simulink library "buildingEnergyComposite"  (R2025b)
settings: Solver=VariableStepAuto  StartTime=0.0  StopTime=10.0  RelTol=1e-3
libraries: fl_lib x59, buildingEnergy_lib x9, SimscapeFluids_lib x1
settings Model: Creator=vikrants  LastModifiedBy=skota

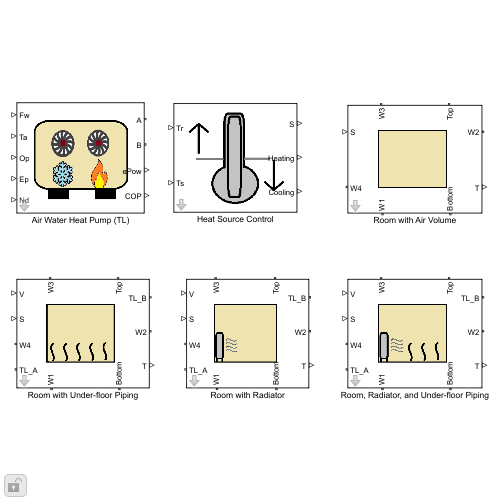
[thumbnail: Simulink's stored preview of the top-level diagram]
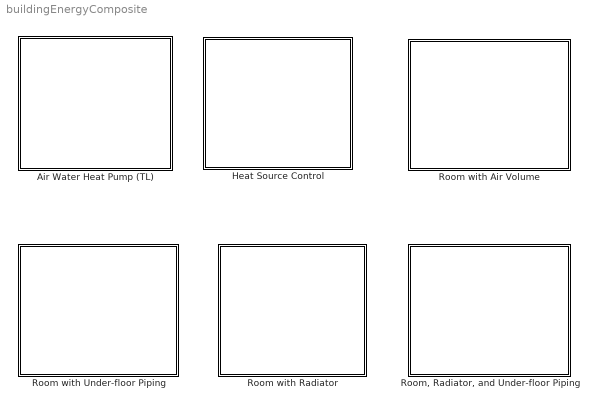
== system buildingEnergyComposite ==
  Air Water Heat Pump (TL) : Subsystem  mask{heatingCapacityA=10.17, heatingCoPA=4.86, heatingCapacityB=10.12, heatingCoPB=3.7, heatingCapacityC=10.17, heatingCoPC=4.86, heatingCapacityD=10.12, heatingCoPD=3.7, coolingCapacityE=10.55, coolingCoPE=4.13, coolingCapacityF=6.9, coolingCoPF=2.7, elecHeaterPower=0, coilLen=2, coilArea=pi*(5e-2^2)/4, coilDia=5e-2, tankVolume=5, initialT=299.8, waterOpTempMax=330, waterOpTempMin=278, initialP=0.101325, measTimelagWater=60, minWaterFlowRate=1e-3, nomFlowDuringTest=0.5}
      mask prompts: heatingCapacityA "A-2W55, estimated heating capacity (kW)"; heatingCoPA "A-2W55, estimated COP (or SCOP)"; heatingCapacityB "A-2W65, estimated heating capacity (kW)"; heatingCoPB "A-2W65, estimated COP (or SCOP)"; heatingCapacityC "A7W35, estimated heating capacity (kW)"; heatingCoPC "A7W35, estimated COP (or SCOP)"; heatingCapacityD "A7W45, estimated heating capacity (kW)"; heatingCoPD "A7W45, estimated COP (or SCOP)"; coolingCapacityE "A35W18, estimated cooling capacity (kW)"; coolingCoPE "A35W18, estimated COP (or SCOP)"; coolingCapacityF "A35W7, estimated cooling capacity (kW)"; coolingCoPF "A35W7, estimated COP (or SCOP)"; elecHeaterPower "Additional electric heater rating (kW)"; coilLen "Length of coil pipe (m)"; coilArea "Area of coil pipe (m^2)"; coilDia "Diameter of coil pipe (m)"; tankVolume "Heat exchanger internal volume (m^3)"; initialT "Initial Temperature (K)"; waterOpTempMax "Maximum operational water temperature"; waterOpTempMin "Minimum operation water temperature"; initialP "Initial pressure of coil pipe water (MPa)"; measTimelagWater "Temperature sensor delay for water flow (s)"; minWaterFlowRate "Minimum water flowrate (kg/s)"; nomFlowDuringTest "Nominal water flowrate during test (kg/s)"
      mask Help: web("DocumentationAirWaterHeatPumpTL.html")
      mask DialogControl DescGroupVar Prompt: Description
      mask DialogControl DescTextVar Prompt: Heat pump model based on EN14511 test data.
      mask DialogControl Container3 Prompt: EN14511 (Heating) Data
      mask DialogControl Container4 Prompt: EN14511 (Cooling) Data
      mask DialogControl ParameterGroupVar Prompt: Heat Pump Construction
      mask DialogControl Container5 Prompt: Flow and Thermal Specifications
      mask Display: image('AirWaterHeatPumpTL.png');
  Heat Source Control : Subsystem  mask{capacity=12000, num=1, delT=10, tau=1, iniT=280}
      mask prompts: capacity "Heat pump capacity (W)"; num "Number of sources (-)"; delT "Change in water temperature (deg C)"; tau "Measurement time constant (s)"; iniT "Initial water temperature (K)"
      mask Help: web("DocumentationCompositeHeatSourceControl.html")
      mask DialogControl DescGroupVar Prompt: Description
      mask DialogControl DescTextVar Prompt: The block evaluates heating or cooling requirements for a building  based on the measured room temperatures and the specified set point temperature.
      mask DialogControl HeatPump Prompt: Heat Pump
      mask Display: image('HeatSourceControlIcon.png');
  Room with Air Volume : Subsystem  mask{roomWid=3, roomHgt=2.5, roomLen=5, htc=10, iniT=300, indxS=1}
      mask prompts: roomWid "Room Width (m)"; roomHgt "Room Height (m)"; roomLen "Room Length (m)"; htc "Heat Transfer Coefficient (W/K*m^2)"; iniT "Initial Temperature (K)"; indxS "Heat source vector index"
      settings: PortSchema="{\"entries\":[{\"content\":{\"sides\":[{\"content\":{\"connectorIds\":[\"LConn1\",\"LConn2\"]},\"type\":\"ConnectorPlacement.EquallySpacedRectSide\",\"uuid\":\"8440f6ae-3089-4f14-af97-f7a7d9c670fb\"},{\"content\":{\"connectorIds\":[\"RConn1\",\"RConn2\"],\"side\":\"RIGHT\"},\"type\":\"ConnectorPlacement.EquallySpacedRectSide\",\"uuid\":\"df84a625-bd6d-46a4-b71c-d411d28f8df6\"},{\"content\":{\"connectorIds\":[\"LConn3\",\"LConn4\"],\"side\":\"TOP\"},\"type\":\"ConnectorPlacement.EquallySpacedRectSide\",\"uuid\":\"90f16a0a-d00c-4f13-8e79-f2f23ea8b565\"},{\"content\":{\"connectorIds\":[\"RConn3\",\"RConn4\"],\"side\":\"BOTTOM\"},\"type\":\"ConnectorPlacement.EquallySpacedRectSide\",\"uuid\":\"4eb9d9d9-e9b4-43a3-a1e1-726815f3b9ff\"}]},\"type\":\"ConnectorPlacement.EquallySpacedConnector\",\"uuid\":\"51dc529f-94b8-407e-b287-301b2c0c8383\"}],\"packageUris\":[\"http://schema.mathworks.com/mf0/Connector/R2020b\"],\"version\":\"1.0\"}"
      mask Help: web("DocumentationCompositeRoom.html")
      mask DialogControl DescGroupVar Prompt: Description
      mask DialogControl DescTextVar Prompt: Room model with air volume.
      mask DialogControl ParameterGroupRoom Prompt: Room Dimensions
      mask DialogControl ParameterGroupHT Prompt: Heat Transfer
      mask Display: image("roomWithAirVolume.png");
  Room with Radiator : Subsystem  mask{pipeRoughnessR=1e-6, pipeLenR=10, pipeCrossSectionalAreaR=1.75e-4, pipeHydrDiaR=1.5e-2, roomWid=3, roomHgt=2.5, roomLen=5, htc=10, iniT=300, indxS=1, indxV=1}
      mask prompts: pipeRoughnessR "Pipe roughness (m)"; pipeLenR "Pipe length (m)"; pipeCrossSectionalAreaR "Pipe cross-sectional area (m^2)"; pipeHydrDiaR "Pipe hydraulic diameter (m)"; roomWid "Room Width (m)"; roomHgt "Room Height (m)"; roomLen "Room Length (m)"; htc "Heat Transfer Coefficient (W/K*m^2)"; iniT "Initial Temperature (K)"; indxS "Heat source vector index"; indxV "Valve operation vector index"
      settings: PortSchema="{\"entries\":[{\"content\":{\"sides\":[{\"content\":{\"connectorIds\":[\"LConn1\",\"LConn2\",\"LConn3\",\"LConn4\"]},\"type\":\"ConnectorPlacement.EquallySpacedRectSide\",\"uuid\":\"8440f6ae-3089-4f14-af97-f7a7d9c670fb\"},{\"content\":{\"connectorIds\":[\"RConn1\",\"RConn2\",\"RConn3\"],\"side\":\"RIGHT\"},\"type\":\"ConnectorPlacement.EquallySpacedRectSide\",\"uuid\":\"df84a625-bd6d-46a4-b71c-d411d28f8df6\"},{\"content\":{\"connectorIds\":[\"LConn5\",\"LConn6\"],\"side\":\"TOP\"},\"type\":\"ConnectorPlacement.EquallySpacedRectSide\",\"uuid\":\"90f16a0a-d00c-4f13-8e79-f2f23ea8b565\"},{\"content\":{\"connectorIds\":[\"RConn4\",\"RConn5\"],\"side\":\"BOTTOM\"},\"type\":\"ConnectorPlacement.EquallySpacedRectSide\",\"uuid\":\"4eb9d9d9-e9b4-43a3-a1e1-726815f3b9ff\"}]},\"type\":\"ConnectorPlacement.EquallySpacedConnector\",\"uuid\":\"51dc529f-94b8-407e-b287-301b2c0c8383\"}],\"packageUris\":[\"http://schema.mathworks.com/mf0/Connector/R2020b\"],\"version\":\"1.0\"}"
      mask Help: web("DocumentationCompositeRoomRadiator.html")
      mask DialogControl DescGroupVar Prompt: Description
      mask DialogControl DescTextVar Prompt: Room model with radiator for thermal comfort.
      mask DialogControl ParameterGroupRadiator Prompt: Radiator
      mask DialogControl ParameterGroupRoom Prompt: Room Dimensions
      mask DialogControl ParameterGroupHT Prompt: Heat Transfer
      mask Display: image("roomWithRadiator.png");
  Room with Under-floor Piping : Subsystem  mask{pipeRoughnessUFP=1e-6, pipeLenUFP=50, pipeCrossSectionalAreaUFP=1.75e-4, pipeHydrDiaUFP=1.5e-2, thermalResFloor=100, roomWid=3, roomHgt=2.5, roomLen=5, htc=10, iniT=300, indxS=1, indxV=1}
      mask prompts: pipeRoughnessUFP "Pipe roughness (m)"; pipeLenUFP "Pipe length (m)"; pipeCrossSectionalAreaUFP "Pipe cross-sectional area (m^2)"; pipeHydrDiaUFP "Pipe hydraulic diameter (m)"; thermalResFloor "Thermal resistance to floor (K/W)"; roomWid "Room Width (m)"; roomHgt "Room Height (m)"; roomLen "Room Length (m)"; htc "Heat Transfer Coefficient (W/K*m^2)"; iniT "Initial Temperature (K)"; indxS "Heat source vector index"; indxV "Valve operation vector index"
      settings: PortSchema="{\"entries\":[{\"content\":{\"sides\":[{\"content\":{\"connectorIds\":[\"LConn1\",\"LConn2\",\"LConn3\",\"LConn4\"]},\"type\":\"ConnectorPlacement.EquallySpacedRectSide\",\"uuid\":\"8440f6ae-3089-4f14-af97-f7a7d9c670fb\"},{\"content\":{\"connectorIds\":[\"RConn1\",\"RConn2\",\"RConn3\"],\"side\":\"RIGHT\"},\"type\":\"ConnectorPlacement.EquallySpacedRectSide\",\"uuid\":\"df84a625-bd6d-46a4-b71c-d411d28f8df6\"},{\"content\":{\"connectorIds\":[\"LConn5\",\"LConn6\"],\"side\":\"TOP\"},\"type\":\"ConnectorPlacement.EquallySpacedRectSide\",\"uuid\":\"90f16a0a-d00c-4f13-8e79-f2f23ea8b565\"},{\"content\":{\"connectorIds\":[\"RConn4\",\"RConn5\"],\"side\":\"BOTTOM\"},\"type\":\"ConnectorPlacement.EquallySpacedRectSide\",\"uuid\":\"4eb9d9d9-e9b4-43a3-a1e1-726815f3b9ff\"}]},\"type\":\"ConnectorPlacement.EquallySpacedConnector\",\"uuid\":\"51dc529f-94b8-407e-b287-301b2c0c8383\"}],\"packageUris\":[\"http://schema.mathworks.com/mf0/Connector/R2020b\"],\"version\":\"1.0\"}"
      mask Help: web("DocumentationCompositeRoomUFP.html")
      mask DialogControl DescGroupVar Prompt: Description
      mask DialogControl DescTextVar Prompt: Room model with under-floor piping for thermal comfort.
      mask DialogControl ParameterGroupUFP Prompt: Under Floor Piping
      mask DialogControl ParameterGroupRoom Prompt: Room Dimensions
      mask DialogControl ParameterGroupHT Prompt: Heat Transfer
      mask Display: image("roomWithUFP.png");
  "Room, Radiator, and Under-floor Piping" : Subsystem  mask{pipeRoughnessR=1e-6, pipeLenR=10, pipeCrossSectionalAreaR=1.75e-4, pipeHydrDiaR=1.5e-2, pipeRoughnessUFP=1e-6, pipeLenUFP=50, pipeCrossSectionalAreaUFP=1.75e-4, pipeHydrDiaUFP=1.5e-2, thermalResFloor=100, roomWid=3, roomHgt=2.5, roomLen=5, htc=10, iniT=300, indxS=1, indxV=1}
      mask prompts: pipeRoughnessR "Pipe roughness (m)"; pipeLenR "Pipe length (m)"; pipeCrossSectionalAreaR "Pipe cross-sectional area (m^2)"; pipeHydrDiaR "Pipe hydraulic diameter (m)"; pipeRoughnessUFP "Pipe roughness (m)"; pipeLenUFP "Pipe length (m)"; pipeCrossSectionalAreaUFP "Pipe cross-sectional area (m^2)"; pipeHydrDiaUFP "Pipe hydraulic diameter (m)"; thermalResFloor "Thermal resistance to floor (K/W)"; roomWid "Room Width (m)"; roomHgt "Room Height (m)"; roomLen "Room Length (m)"; htc "Heat Transfer Coefficient (W/K*m^2)"; iniT "Initial Temperature (K)"; indxS "Heat source vector index"; indxV "Valve operation vector index"
      settings: PortSchema="{\"entries\":[{\"content\":{\"sides\":[{\"content\":{\"connectorIds\":[\"LConn1\",\"LConn2\",\"LConn3\",\"LConn4\"]},\"type\":\"ConnectorPlacement.EquallySpacedRectSide\",\"uuid\":\"8440f6ae-3089-4f14-af97-f7a7d9c670fb\"},{\"content\":{\"connectorIds\":[\"RConn1\",\"RConn2\",\"RConn3\"],\"side\":\"RIGHT\"},\"type\":\"ConnectorPlacement.EquallySpacedRectSide\",\"uuid\":\"df84a625-bd6d-46a4-b71c-d411d28f8df6\"},{\"content\":{\"connectorIds\":[\"LConn5\",\"LConn6\"],\"side\":\"TOP\"},\"type\":\"ConnectorPlacement.EquallySpacedRectSide\",\"uuid\":\"90f16a0a-d00c-4f13-8e79-f2f23ea8b565\"},{\"content\":{\"connectorIds\":[\"RConn4\",\"RConn5\"],\"side\":\"BOTTOM\"},\"type\":\"ConnectorPlacement.EquallySpacedRectSide\",\"uuid\":\"4eb9d9d9-e9b4-43a3-a1e1-726815f3b9ff\"}]},\"type\":\"ConnectorPlacement.EquallySpacedConnector\",\"uuid\":\"51dc529f-94b8-407e-b287-301b2c0c8383\"}],\"packageUris\":[\"http://schema.mathworks.com/mf0/Connector/R2020b\"],\"version\":\"1.0\"}"
      mask Help: web("DocumentationCompositeRoomRadiatorUFP.html")
      mask DialogControl DescGroupVar Prompt: Description
      mask DialogControl DescTextVar Prompt: Room model with radiator and under-floor piping for thermal comfort.
      mask DialogControl ParameterGroupRadiator Prompt: Radiator
      mask DialogControl ParameterGroupUFP Prompt: Under Floor Piping
      mask DialogControl ParameterGroupRoom Prompt: Room Dimensions
      mask DialogControl ParameterGroupHT Prompt: Heat Transfer
      mask Display: image("roomWithRadiatorAndUFP.png");

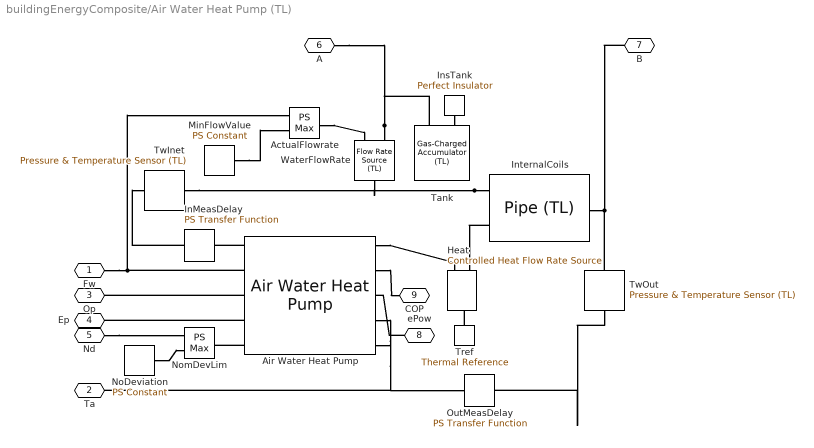
== system buildingEnergyComposite/Air Water Heat Pump (TL) ==
  ActualFlowrate : fl_lib/Physical Signals/Nonlinear Operators/PS Max  ZeroCross=true
  Air Water Heat Pump : buildingEnergy_lib/Air Water Heat Pump  nominalCapacityA=heatingCapacityA kW  seasonalCOPvalA=heatingCoPA  nominalCapacityB=heatingCapacityB kW  seasonalCOPvalB=heatingCoPB  nominalCapacityC=heatingCapacityC kW  seasonalCOPvalC=heatingCoPC  nominalCapacityD=heatingCapacityD kW  seasonalCOPvalD=heatingCoPD  nominalCapacityE=coolingCapacityE kW  seasonalCOPvalE=coolingCoPE  nominalCapacityF=coolingCapacityF kW  seasonalCOPvalF=coolingCoPF  backupElecHeater=elecHeaterPower kW  wInletOpRangeUpp=waterOpTempMax K  wInletOpRangeLow=waterOpTempMin K  airTemperatureVector=273 + [-2, -2, 7, 7, 35, 35]  waterTemperatureVector=273 + [55, 65, 35, 45, 18, 7]  waterSpHeat=4186 J/(K*kg)  smallPower=1e-3 W  maxCOP_specify=off  maxCOP_priority=None  maxCOP=8  maxCOP_nominal_specify=off  maxCOP_nominal_value=1  maxCOP_nominal_unit=1
  Heat : fl_lib/Thermal/Thermal Sources/Controlled Heat Flow Rate Source
  InMeasDelay : fl_lib/Physical Signals/Linear Operators/PS Transfer Function  transfer_function_type=foundation.enum.transfer_function_type.lag  T=measTimelagWater s  T1=2 s  T2=1 s  reset_method=foundation.enum.IntegratorResetSpec.None  initial_condition_spec=foundation.enum.IntegratorICSpec.Internal  y0=initialT K
  InsTank : fl_lib/Thermal/Thermal Elements/Perfect Insulator  T_specify=off  T_priority=None  T=293.15 K  T_nominal_specify=off  T_nominal_value=1  T_nominal_unit=K
  InternalCoils : fl_lib/Thermal Liquid/Elements/Pipe (TL)  length=coilLen m  area=coilArea m^2  Dh=coilDia m  length_add=0 m  roughness=15e-6 m  Re_lam=2000  Re_tur=4000  shape_factor=64  Nu_lam=3.66  dynamic_compressibility=true  inertia=false  p0=initialP MPa  T0=initialT K  mdot0=0 kg/s  p_nominal=0.101325 MPa  T_nominal=293.15 K
  MinFlowValue : fl_lib/Physical Signals/Sources/PS Constant  constant=minWaterFlowRate kg/s
  NoDeviation : fl_lib/Physical Signals/Sources/PS Constant  constant=1
  NomDevLim : fl_lib/Physical Signals/Nonlinear Operators/PS Max  ZeroCross=true
  OutMeasDelay : fl_lib/Physical Signals/Linear Operators/PS Transfer Function  transfer_function_type=foundation.enum.transfer_function_type.lag  T=measTimelagWater s  T1=2 s  T2=1 s  reset_method=foundation.enum.IntegratorResetSpec.None  initial_condition_spec=foundation.enum.IntegratorICSpec.Internal  y0=initialT K
  Tank : SimscapeFluids_lib/Thermal Liquid/Tanks & Accumulators/Gas-Charged Accumulator (TL)  capacity=tankVolume m^3  dead_volume=4e-5 m^3  p_precharge_gauge=0 MPa  k_sh=1.4  area=0.01 m^2  stiff_coeff=1e4 MPa/m^3  damping_coeff=1e4 MPa*s/m^6  liquid_volume_specify=off  liquid_volume_priority=High  liquid_volume=5e-3 m^3  liquid_volume_nominal_specify=off  liquid_volume_nominal_value=1  liquid_volume_nominal_unit=m^3  liquid_mass_specify=off  liquid_mass_priority=None  liquid_mass=5 kg  liquid_mass_nominal_specify=off  liquid_mass_nominal_value=1  liquid_mass_nominal_unit=kg  p_I_specify=off  p_I_priority=None  p_I=0.101325 MPa  p_I_nominal_specify=off  p_I_nominal_value=1  p_I_nominal_unit=MPa  T_I_specify=on  T_I_priority=High  T_I=initialT K  T_I_nominal_specify=off  T_I_nominal_value=1  T_I_nominal_unit=K
  Tref : fl_lib/Thermal/Thermal Elements/Thermal Reference
  TwInet : fl_lib/Thermal Liquid/Sensors/Pressure & Temperature Sensor (TL)  reference=foundation.enum.MeasurementReference.absolute  pressure=false  pressure_spec=foundation.enum.PressureMeasementSpec.Absolute  temperature=true
  TwOut : fl_lib/Thermal Liquid/Sensors/Pressure & Temperature Sensor (TL)  reference=foundation.enum.MeasurementReference.absolute  pressure=false  pressure_spec=foundation.enum.PressureMeasementSpec.Absolute  temperature=true
  WaterFlowRate : fl_lib/Thermal Liquid/Sources/Flow Rate Source (TL)  source_type=foundation.enum.constant_controlled.controlled  flow_type=foundation.enum.mass_volumetric_flow.mass  mass_flow=0 kg/s  volumetric_flow=0 m^3/s  power_spec=foundation.enum.power_spec.none  area=coilArea m^2
  Fw : PMIOPort  Side=Left
  Ta : PMIOPort  Port=2  Side=Left
  Op : PMIOPort  Port=3  Side=Left
  Ep : PMIOPort  Port=4  Side=Left
  Nd : PMIOPort  Port=5  Side=Left
  A : PMIOPort  Port=6  Side=Right
  B : PMIOPort  Port=7  Side=Right
  ePow : PMIOPort  Port=8  Side=Right
  COP : PMIOPort  Port=9  Side=Right
  connections:
  TwOut/LConn1 -- B/RConn1 -- InternalCoils/RConn1
  InternalCoils/LConn1 -- WaterFlowRate/RConn1 -- TwInet/LConn1
  Fw/RConn1 -- Air Water Heat Pump/LConn2 -- ActualFlowrate/LConn1
  WaterFlowRate/LConn1 -- A/RConn1 -- Tank/RConn1
  Air Water Heat Pump/LConn1 -- InMeasDelay/RConn1
  Air Water Heat Pump/LConn3 -- Op/RConn1
  InMeasDelay/LConn1 -- TwInet/RConn1
  InternalCoils/LConn2 -- Heat/RConn2
  ePow/RConn1 -- Air Water Heat Pump/RConn3
  InsTank/LConn1 -- Tank/RConn2
  NoDeviation/RConn1 -- NomDevLim/LConn2
  Air Water Heat Pump/LConn4 -- Ep/RConn1
  Air Water Heat Pump/RConn2 -- COP/RConn1
  ActualFlowrate/RConn1 -- WaterFlowRate/LConn2
  MinFlowValue/RConn1 -- ActualFlowrate/LConn2
  Air Water Heat Pump/RConn5 -- OutMeasDelay/RConn1
  Tref/LConn1 -- Heat/LConn1
  Air Water Heat Pump/LConn5 -- NomDevLim/RConn1
  TwOut/RConn1 -- OutMeasDelay/LConn1
  Nd/RConn1 -- NomDevLim/LConn1
  Air Water Heat Pump/RConn4 -- Ta/RConn1
  Air Water Heat Pump/RConn1 -- Heat/RConn1

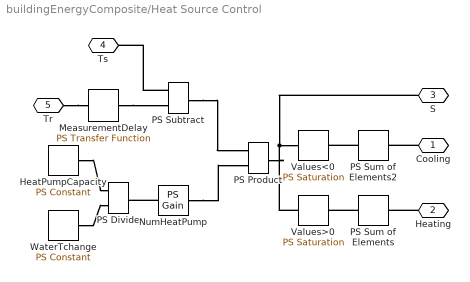
== system buildingEnergyComposite/Heat Source Control ==
  HeatPumpCapacity : fl_lib/Physical Signals/Sources/PS Constant  constant=capacity J/s
  MeasurementDelay : fl_lib/Physical Signals/Linear Operators/PS Transfer Function  transfer_function_type=foundation.enum.transfer_function_type.lag  T=tau s  T1=2 s  T2=1 s  reset_method=foundation.enum.IntegratorResetSpec.None  initial_condition_spec=foundation.enum.IntegratorICSpec.Internal  y0=iniT K
  NumHeatPump : fl_lib/Physical Signals/Functions/PS Gain  gain=num
  PS Divide : fl_lib/Physical Signals/Functions/PS Divide
  PS Product : fl_lib/Physical Signals/Functions/PS Product
  PS Subtract : fl_lib/Physical Signals/Functions/PS Subtract
  PS Sum of Elements : fl_lib/Physical Signals/Functions/PS Sum of Elements  sumAll=true
  PS Sum of Elements2 : fl_lib/Physical Signals/Functions/PS Sum of Elements  sumAll=true
  Values<0 : fl_lib/Physical Signals/Nonlinear Operators/PS Saturation  upper_limit=0 J/s  lower_limit=-inf J/s  ZeroCross=true
  Values>0 : fl_lib/Physical Signals/Nonlinear Operators/PS Saturation  upper_limit=inf J/s  lower_limit=0 J/s  ZeroCross=true
  WaterTchange : fl_lib/Physical Signals/Sources/PS Constant  constant=delT K
  Cooling : PMIOPort  Side=Left
  Heating : PMIOPort  Port=2  Side=Left
  S : PMIOPort  Port=3  Side=Left
  Ts : PMIOPort  Port=4  Side=Right
  Tr : PMIOPort  Port=5  Side=Right
  connections:
  PS Subtract/RConn1 -- PS Product/LConn1
  Tr/RConn1 -- MeasurementDelay/LConn1
  PS Subtract/LConn1 -- Ts/RConn1
  Heating/RConn1 -- PS Sum of Elements/RConn1
  Cooling/RConn1 -- PS Sum of Elements2/RConn1
  PS Sum of Elements/LConn1 -- Values>0/RConn1
  PS Sum of Elements2/LConn1 -- Values<0/RConn1
  MeasurementDelay/RConn1 -- PS Subtract/LConn2
  HeatPumpCapacity/RConn1 -- PS Divide/LConn1
  WaterTchange/RConn1 -- PS Divide/LConn2
  NumHeatPump/LConn1 -- PS Divide/RConn1
  NumHeatPump/RConn1 -- PS Product/LConn2
  S/RConn1 -- Values<0/LConn1 -- Values>0/LConn1 -- PS Product/RConn1

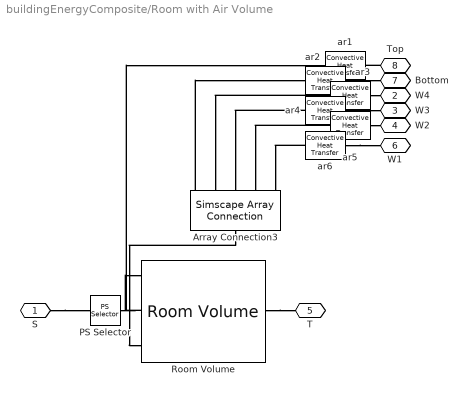
== system buildingEnergyComposite/Room with Air Volume ==
  Array Connection3 : SimscapeArrayConnection  Domain=foundation.thermal.thermal  NumScalarElements=5
  PS Selector : fl_lib/Physical Signals/Nonlinear Operators/PS Selector  ix=indxS
  Room Volume : buildingEnergy_lib/Room Volume  N1=1  N2=5  iniT=iniT K  length=roomLen m  width=roomWid m  height=roomHgt m
  ar1 : fl_lib/Thermal/Thermal Elements/Convective Heat Transfer  thermal_type=foundation.enum.constant_variable.constant  area=roomLen*roomWid m^2  heat_tr_coeff=htc W/(K*m^2)  min_heat_tr_coeff=1e-3 W/(K*m^2)  T_specify=off  T_priority=None  T=0 K  T_nominal_specify=off  T_nominal_value=1  T_nominal_unit=K  Q_specify=off  Q_priority=None  Q=0 W  Q_nominal_specify=off  Q_nominal_value=1  Q_nominal_unit=W
  ar2 : fl_lib/Thermal/Thermal Elements/Convective Heat Transfer  thermal_type=foundation.enum.constant_variable.constant  area=roomLen*roomWid m^2  heat_tr_coeff=htc W/(K*m^2)  min_heat_tr_coeff=1e-3 W/(K*m^2)  T_specify=off  T_priority=None  T=0 K  T_nominal_specify=off  T_nominal_value=1  T_nominal_unit=K  Q_specify=off  Q_priority=None  Q=0 W  Q_nominal_specify=off  Q_nominal_value=1  Q_nominal_unit=W
  ar3 : fl_lib/Thermal/Thermal Elements/Convective Heat Transfer  thermal_type=foundation.enum.constant_variable.constant  area=roomHgt*roomWid m^2  heat_tr_coeff=htc W/(K*m^2)  min_heat_tr_coeff=1e-3 W/(K*m^2)  T_specify=off  T_priority=None  T=0 K  T_nominal_specify=off  T_nominal_value=1  T_nominal_unit=K  Q_specify=off  Q_priority=None  Q=0 W  Q_nominal_specify=off  Q_nominal_value=1  Q_nominal_unit=W
  ar4 : fl_lib/Thermal/Thermal Elements/Convective Heat Transfer  thermal_type=foundation.enum.constant_variable.constant  area=roomLen*roomHgt m^2  heat_tr_coeff=htc W/(K*m^2)  min_heat_tr_coeff=1e-3 W/(K*m^2)  T_specify=off  T_priority=None  T=0 K  T_nominal_specify=off  T_nominal_value=1  T_nominal_unit=K  Q_specify=off  Q_priority=None  Q=0 W  Q_nominal_specify=off  Q_nominal_value=1  Q_nominal_unit=W
  ar5 : fl_lib/Thermal/Thermal Elements/Convective Heat Transfer  thermal_type=foundation.enum.constant_variable.constant  area=roomHgt*roomWid m^2  heat_tr_coeff=htc W/(K*m^2)  min_heat_tr_coeff=1e-3 W/(K*m^2)  T_specify=off  T_priority=None  T=0 K  T_nominal_specify=off  T_nominal_value=1  T_nominal_unit=K  Q_specify=off  Q_priority=None  Q=0 W  Q_nominal_specify=off  Q_nominal_value=1  Q_nominal_unit=W
  ar6 : fl_lib/Thermal/Thermal Elements/Convective Heat Transfer  thermal_type=foundation.enum.constant_variable.constant  area=roomLen*roomHgt m^2  heat_tr_coeff=htc W/(K*m^2)  min_heat_tr_coeff=1e-3 W/(K*m^2)  T_specify=off  T_priority=None  T=0 K  T_nominal_specify=off  T_nominal_value=1  T_nominal_unit=K  Q_specify=off  Q_priority=None  Q=0 W  Q_nominal_specify=off  Q_nominal_value=1  Q_nominal_unit=W
  S : PMIOPort  Side=Left
  W4 : PMIOPort  Port=2  Side=Left
  W3 : PMIOPort  Port=3  Side=Left
  W2 : PMIOPort  Port=4  Side=Right
  T : PMIOPort  Port=5  Side=Right
  W1 : PMIOPort  Port=6  Side=Right
  Bottom : PMIOPort  Port=7  Side=Right
  Top : PMIOPort  Port=8  Side=Left
  connections:
  Array Connection3/RConn1 -- Room Volume/LConn3
  Room Volume/RConn1 -- T/RConn1
  ar6/RConn1 -- W1/RConn1
  ar5/RConn1 -- W2/RConn1
  ar4/RConn1 -- W3/RConn1
  ar3/RConn1 -- W4/RConn1
  Top/RConn1 -- ar1/RConn1
  ar2/RConn1 -- Bottom/RConn1
  Array Connection3/LConn1 -- ar2/LConn1
  ar3/LConn1 -- Array Connection3/LConn2
  ar4/LConn1 -- Array Connection3/LConn3
  ar5/LConn1 -- Array Connection3/LConn4
  ar6/LConn1 -- Array Connection3/LConn5
  PS Selector/RConn1 -- Room Volume/LConn1
  S/RConn1 -- PS Selector/LConn1
  Room Volume/LConn2 -- ar1/LConn1

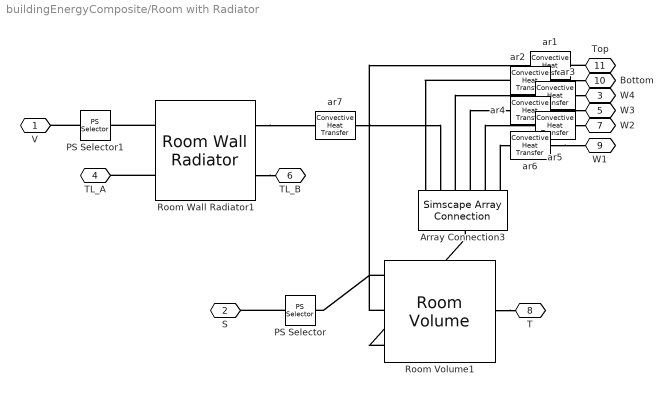
== system buildingEnergyComposite/Room with Radiator ==
  Array Connection3 : SimscapeArrayConnection  Domain=foundation.thermal.thermal  NumScalarElements=6
  PS Selector : fl_lib/Physical Signals/Nonlinear Operators/PS Selector  ix=indxS
  PS Selector1 : fl_lib/Physical Signals/Nonlinear Operators/PS Selector  ix=indxV
  Room Volume1 : buildingEnergy_lib/Room Volume  N1=1  N2=6  iniT=iniT K  length=roomLen m  width=roomWid m  height=roomHgt m
  Room Wall Radiator1 : buildingEnergy_lib/Room Wall Radiator  pipeHydrDia=pipeHydrDiaR m  pipeLength=pipeLenR m  pipeArea=pipeCrossSectionalAreaR m^2  pipeRoughness=pipeRoughnessR m  htc=htc W/(K*m^2)  iniTemperature=iniT K
  ar1 : fl_lib/Thermal/Thermal Elements/Convective Heat Transfer  thermal_type=foundation.enum.constant_variable.constant  area=roomLen*roomWid m^2  heat_tr_coeff=htc W/(K*m^2)  min_heat_tr_coeff=1e-3 W/(K*m^2)  T_specify=off  T_priority=None  T=0 K  T_nominal_specify=off  T_nominal_value=1  T_nominal_unit=K  Q_specify=off  Q_priority=None  Q=0 W  Q_nominal_specify=off  Q_nominal_value=1  Q_nominal_unit=W
  ar2 : fl_lib/Thermal/Thermal Elements/Convective Heat Transfer  thermal_type=foundation.enum.constant_variable.constant  area=roomLen*roomWid m^2  heat_tr_coeff=htc W/(K*m^2)  min_heat_tr_coeff=1e-3 W/(K*m^2)  T_specify=off  T_priority=None  T=0 K  T_nominal_specify=off  T_nominal_value=1  T_nominal_unit=K  Q_specify=off  Q_priority=None  Q=0 W  Q_nominal_specify=off  Q_nominal_value=1  Q_nominal_unit=W
  ar3 : fl_lib/Thermal/Thermal Elements/Convective Heat Transfer  thermal_type=foundation.enum.constant_variable.constant  area=roomHgt*roomWid m^2  heat_tr_coeff=htc W/(K*m^2)  min_heat_tr_coeff=1e-3 W/(K*m^2)  T_specify=off  T_priority=None  T=0 K  T_nominal_specify=off  T_nominal_value=1  T_nominal_unit=K  Q_specify=off  Q_priority=None  Q=0 W  Q_nominal_specify=off  Q_nominal_value=1  Q_nominal_unit=W
  ar4 : fl_lib/Thermal/Thermal Elements/Convective Heat Transfer  thermal_type=foundation.enum.constant_variable.constant  area=roomLen*roomHgt m^2  heat_tr_coeff=htc W/(K*m^2)  min_heat_tr_coeff=1e-3 W/(K*m^2)  T_specify=off  T_priority=None  T=0 K  T_nominal_specify=off  T_nominal_value=1  T_nominal_unit=K  Q_specify=off  Q_priority=None  Q=0 W  Q_nominal_specify=off  Q_nominal_value=1  Q_nominal_unit=W
  ar5 : fl_lib/Thermal/Thermal Elements/Convective Heat Transfer  thermal_type=foundation.enum.constant_variable.constant  area=roomHgt*roomWid m^2  heat_tr_coeff=htc W/(K*m^2)  min_heat_tr_coeff=1e-3 W/(K*m^2)  T_specify=off  T_priority=None  T=0 K  T_nominal_specify=off  T_nominal_value=1  T_nominal_unit=K  Q_specify=off  Q_priority=None  Q=0 W  Q_nominal_specify=off  Q_nominal_value=1  Q_nominal_unit=W
  ar6 : fl_lib/Thermal/Thermal Elements/Convective Heat Transfer  thermal_type=foundation.enum.constant_variable.constant  area=roomLen*roomHgt m^2  heat_tr_coeff=htc W/(K*m^2)  min_heat_tr_coeff=1e-3 W/(K*m^2)  T_specify=off  T_priority=None  T=0 K  T_nominal_specify=off  T_nominal_value=1  T_nominal_unit=K  Q_specify=off  Q_priority=None  Q=0 W  Q_nominal_specify=off  Q_nominal_value=1  Q_nominal_unit=W
  ar7 : fl_lib/Thermal/Thermal Elements/Convective Heat Transfer  thermal_type=foundation.enum.constant_variable.constant  area=pipeLenR*pipeHydrDiaR m^2  heat_tr_coeff=htc W/(K*m^2)  min_heat_tr_coeff=1e-3 W/(K*m^2)  T_specify=off  T_priority=None  T=0 K  T_nominal_specify=off  T_nominal_value=1  T_nominal_unit=K  Q_specify=off  Q_priority=None  Q=0 W  Q_nominal_specify=off  Q_nominal_value=1  Q_nominal_unit=W
  V : PMIOPort  Side=Left
  S : PMIOPort  Port=2  Side=Left
  W4 : PMIOPort  Port=3  Side=Left
  TL_A : PMIOPort  Port=4  Side=Left
  W3 : PMIOPort  Port=5  Side=Left
  TL_B : PMIOPort  Port=6  Side=Right
  W2 : PMIOPort  Port=7  Side=Right
  T : PMIOPort  Port=8  Side=Right
  W1 : PMIOPort  Port=9  Side=Right
  Bottom : PMIOPort  Port=10  Side=Right
  Top : PMIOPort  Port=11  Side=Left
  connections:
  Room Wall Radiator1/RConn2 -- TL_B/RConn1
  Room Volume1/RConn1 -- T/RConn1
  Room Wall Radiator1/LConn2 -- TL_A/RConn1
  ar6/RConn1 -- W1/RConn1
  ar5/RConn1 -- W2/RConn1
  ar4/RConn1 -- W3/RConn1
  ar3/RConn1 -- W4/RConn1
  ar7/RConn1 -- Array Connection3/LConn2
  Top/RConn1 -- ar1/RConn1
  ar2/RConn1 -- Bottom/RConn1
  Array Connection3/LConn3 -- ar3/LConn1
  Array Connection3/LConn4 -- ar4/LConn1
  Array Connection3/LConn5 -- ar5/LConn1
  Array Connection3/LConn6 -- ar6/LConn1
  Room Wall Radiator1/RConn1 -- ar7/LConn1
  ar2/LConn1 -- Array Connection3/LConn1
  Room Wall Radiator1/LConn1 -- PS Selector1/RConn1
  PS Selector1/LConn1 -- V/RConn1
  PS Selector/LConn1 -- S/RConn1
  Room Volume1/LConn1 -- PS Selector/RConn1
  Room Volume1/LConn3 -- Array Connection3/RConn1
  Room Volume1/LConn2 -- ar1/LConn1

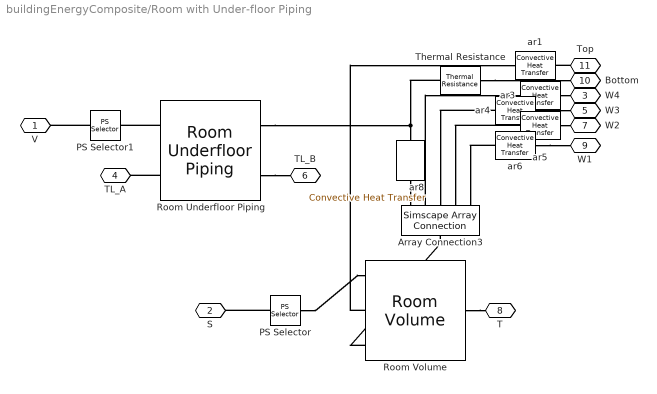
== system buildingEnergyComposite/Room with Under-floor Piping ==
  Array Connection3 : SimscapeArrayConnection  Domain=foundation.thermal.thermal  NumScalarElements=5
  PS Selector : fl_lib/Physical Signals/Nonlinear Operators/PS Selector  ix=indxS
  PS Selector1 : fl_lib/Physical Signals/Nonlinear Operators/PS Selector  ix=indxV
  Room Underfloor Piping : buildingEnergy_lib/Room Underfloor Piping  pipeHydrDia=pipeHydrDiaUFP m  pipeLength=pipeLenUFP m  pipeArea=pipeCrossSectionalAreaUFP m^2  pipeRoughness=pipeRoughnessUFP m  htc=htc W/(K*m^2)  iniTemperature=iniT K
  Room Volume : buildingEnergy_lib/Room Volume  N1=1  N2=5  iniT=iniT K  length=roomLen m  width=roomWid m  height=roomHgt m
  Thermal Resistance : fl_lib/Thermal/Thermal Elements/Thermal Resistance  resistance=thermalResFloor K/W  T_specify=off  T_priority=None  T=0 K  T_nominal_specify=off  T_nominal_value=1  T_nominal_unit=K  Q_specify=off  Q_priority=None  Q=0 W  Q_nominal_specify=off  Q_nominal_value=1  Q_nominal_unit=W
  ar1 : fl_lib/Thermal/Thermal Elements/Convective Heat Transfer  thermal_type=foundation.enum.constant_variable.constant  area=roomLen*roomWid m^2  heat_tr_coeff=htc W/(K*m^2)  min_heat_tr_coeff=1e-3 W/(K*m^2)  T_specify=off  T_priority=None  T=0 K  T_nominal_specify=off  T_nominal_value=1  T_nominal_unit=K  Q_specify=off  Q_priority=None  Q=0 W  Q_nominal_specify=off  Q_nominal_value=1  Q_nominal_unit=W
  ar3 : fl_lib/Thermal/Thermal Elements/Convective Heat Transfer  thermal_type=foundation.enum.constant_variable.constant  area=roomHgt*roomWid m^2  heat_tr_coeff=htc W/(K*m^2)  min_heat_tr_coeff=1e-3 W/(K*m^2)  T_specify=off  T_priority=None  T=0 K  T_nominal_specify=off  T_nominal_value=1  T_nominal_unit=K  Q_specify=off  Q_priority=None  Q=0 W  Q_nominal_specify=off  Q_nominal_value=1  Q_nominal_unit=W
  ar4 : fl_lib/Thermal/Thermal Elements/Convective Heat Transfer  thermal_type=foundation.enum.constant_variable.constant  area=roomLen*roomHgt m^2  heat_tr_coeff=htc W/(K*m^2)  min_heat_tr_coeff=1e-3 W/(K*m^2)  T_specify=off  T_priority=None  T=0 K  T_nominal_specify=off  T_nominal_value=1  T_nominal_unit=K  Q_specify=off  Q_priority=None  Q=0 W  Q_nominal_specify=off  Q_nominal_value=1  Q_nominal_unit=W
  ar5 : fl_lib/Thermal/Thermal Elements/Convective Heat Transfer  thermal_type=foundation.enum.constant_variable.constant  area=roomHgt*roomWid m^2  heat_tr_coeff=htc W/(K*m^2)  min_heat_tr_coeff=1e-3 W/(K*m^2)  T_specify=off  T_priority=None  T=0 K  T_nominal_specify=off  T_nominal_value=1  T_nominal_unit=K  Q_specify=off  Q_priority=None  Q=0 W  Q_nominal_specify=off  Q_nominal_value=1  Q_nominal_unit=W
  ar6 : fl_lib/Thermal/Thermal Elements/Convective Heat Transfer  thermal_type=foundation.enum.constant_variable.constant  area=roomLen*roomHgt m^2  heat_tr_coeff=htc W/(K*m^2)  min_heat_tr_coeff=1e-3 W/(K*m^2)  T_specify=off  T_priority=None  T=0 K  T_nominal_specify=off  T_nominal_value=1  T_nominal_unit=K  Q_specify=off  Q_priority=None  Q=0 W  Q_nominal_specify=off  Q_nominal_value=1  Q_nominal_unit=W
  ar8 : fl_lib/Thermal/Thermal Elements/Convective Heat Transfer  thermal_type=foundation.enum.constant_variable.constant  area=pipeLenUFP*pipeHydrDiaUFP/2 m^2  heat_tr_coeff=htc W/(K*m^2)  min_heat_tr_coeff=1e-3 W/(K*m^2)  T_specify=off  T_priority=None  T=0 K  T_nominal_specify=off  T_nominal_value=1  T_nominal_unit=K  Q_specify=off  Q_priority=None  Q=0 W  Q_nominal_specify=off  Q_nominal_value=1  Q_nominal_unit=W
  V : PMIOPort  Side=Left
  S : PMIOPort  Port=2  Side=Left
  W4 : PMIOPort  Port=3  Side=Left
  TL_A : PMIOPort  Port=4  Side=Left
  W3 : PMIOPort  Port=5  Side=Left
  TL_B : PMIOPort  Port=6  Side=Right
  W2 : PMIOPort  Port=7  Side=Right
  T : PMIOPort  Port=8  Side=Right
  W1 : PMIOPort  Port=9  Side=Right
  Bottom : PMIOPort  Port=10  Side=Right
  Top : PMIOPort  Port=11  Side=Left
  connections:
  Room Underfloor Piping/LConn2 -- TL_A/RConn1
  Room Underfloor Piping/RConn2 -- TL_B/RConn1
  Room Volume/RConn1 -- T/RConn1
  ar6/RConn1 -- W1/RConn1
  ar5/RConn1 -- W2/RConn1
  ar4/RConn1 -- W3/RConn1
  ar3/RConn1 -- W4/RConn1
  Thermal Resistance/LConn1 -- Room Underfloor Piping/RConn1 -- ar8/LConn1
  Top/RConn1 -- ar1/RConn1
  Thermal Resistance/RConn1 -- Bottom/RConn1
  ar8/RConn1 -- Array Connection3/LConn1
  Array Connection3/LConn2 -- ar3/LConn1
  ar4/LConn1 -- Array Connection3/LConn3
  ar5/LConn1 -- Array Connection3/LConn4
  ar6/LConn1 -- Array Connection3/LConn5
  PS Selector/LConn1 -- S/RConn1
  Room Underfloor Piping/LConn1 -- PS Selector1/RConn1
  PS Selector1/LConn1 -- V/RConn1
  PS Selector/RConn1 -- Room Volume/LConn1
  Room Volume/LConn3 -- Array Connection3/RConn1
  Room Volume/LConn2 -- ar1/LConn1

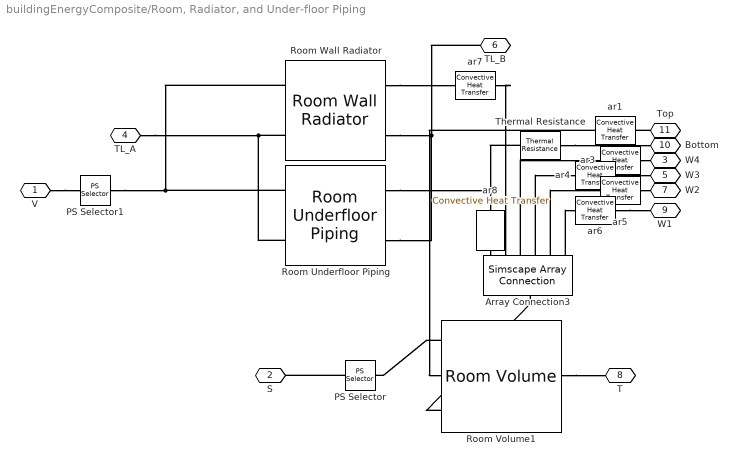
== system buildingEnergyComposite/Room, Radiator, and Under-floor Piping ==
  Array Connection3 : SimscapeArrayConnection  Domain=foundation.thermal.thermal  NumScalarElements=6
  PS Selector : fl_lib/Physical Signals/Nonlinear Operators/PS Selector  ix=indxS
  PS Selector1 : fl_lib/Physical Signals/Nonlinear Operators/PS Selector  ix=indxV
  Room Underfloor Piping : buildingEnergy_lib/Room Underfloor Piping  pipeHydrDia=pipeHydrDiaUFP m  pipeLength=pipeLenUFP m  pipeArea=pipeCrossSectionalAreaUFP m^2  pipeRoughness=pipeRoughnessUFP m  htc=htc W/(K*m^2)  iniTemperature=iniT K
  Room Volume1 : buildingEnergy_lib/Room Volume  N1=1  N2=6  iniT=iniT K  length=roomLen m  width=roomWid m  height=roomHgt m
  Room Wall Radiator : buildingEnergy_lib/Room Wall Radiator  pipeHydrDia=pipeHydrDiaR m  pipeLength=pipeLenR m  pipeArea=pipeCrossSectionalAreaR m^2  pipeRoughness=pipeRoughnessR m  htc=htc W/(K*m^2)  iniTemperature=iniT K
  Thermal Resistance : fl_lib/Thermal/Thermal Elements/Thermal Resistance  resistance=thermalResFloor K/W  T_specify=off  T_priority=None  T=0 K  T_nominal_specify=off  T_nominal_value=1  T_nominal_unit=K  Q_specify=off  Q_priority=None  Q=0 W  Q_nominal_specify=off  Q_nominal_value=1  Q_nominal_unit=W
  ar1 : fl_lib/Thermal/Thermal Elements/Convective Heat Transfer  thermal_type=foundation.enum.constant_variable.constant  area=roomLen*roomWid m^2  heat_tr_coeff=htc W/(K*m^2)  min_heat_tr_coeff=1e-3 W/(K*m^2)  T_specify=off  T_priority=None  T=0 K  T_nominal_specify=off  T_nominal_value=1  T_nominal_unit=K  Q_specify=off  Q_priority=None  Q=0 W  Q_nominal_specify=off  Q_nominal_value=1  Q_nominal_unit=W
  ar3 : fl_lib/Thermal/Thermal Elements/Convective Heat Transfer  thermal_type=foundation.enum.constant_variable.constant  area=roomHgt*roomWid m^2  heat_tr_coeff=htc W/(K*m^2)  min_heat_tr_coeff=1e-3 W/(K*m^2)  T_specify=off  T_priority=None  T=0 K  T_nominal_specify=off  T_nominal_value=1  T_nominal_unit=K  Q_specify=off  Q_priority=None  Q=0 W  Q_nominal_specify=off  Q_nominal_value=1  Q_nominal_unit=W
  ar4 : fl_lib/Thermal/Thermal Elements/Convective Heat Transfer  thermal_type=foundation.enum.constant_variable.constant  area=roomLen*roomHgt m^2  heat_tr_coeff=htc W/(K*m^2)  min_heat_tr_coeff=1e-3 W/(K*m^2)  T_specify=off  T_priority=None  T=0 K  T_nominal_specify=off  T_nominal_value=1  T_nominal_unit=K  Q_specify=off  Q_priority=None  Q=0 W  Q_nominal_specify=off  Q_nominal_value=1  Q_nominal_unit=W
  ar5 : fl_lib/Thermal/Thermal Elements/Convective Heat Transfer  thermal_type=foundation.enum.constant_variable.constant  area=roomHgt*roomWid m^2  heat_tr_coeff=htc W/(K*m^2)  min_heat_tr_coeff=1e-3 W/(K*m^2)  T_specify=off  T_priority=None  T=0 K  T_nominal_specify=off  T_nominal_value=1  T_nominal_unit=K  Q_specify=off  Q_priority=None  Q=0 W  Q_nominal_specify=off  Q_nominal_value=1  Q_nominal_unit=W
  ar6 : fl_lib/Thermal/Thermal Elements/Convective Heat Transfer  thermal_type=foundation.enum.constant_variable.constant  area=roomLen*roomHgt m^2  heat_tr_coeff=htc W/(K*m^2)  min_heat_tr_coeff=1e-3 W/(K*m^2)  T_specify=off  T_priority=None  T=0 K  T_nominal_specify=off  T_nominal_value=1  T_nominal_unit=K  Q_specify=off  Q_priority=None  Q=0 W  Q_nominal_specify=off  Q_nominal_value=1  Q_nominal_unit=W
  ar7 : fl_lib/Thermal/Thermal Elements/Convective Heat Transfer  thermal_type=foundation.enum.constant_variable.constant  area=pipeLenR*pipeHydrDiaR m^2  heat_tr_coeff=htc W/(K*m^2)  min_heat_tr_coeff=1e-3 W/(K*m^2)  T_specify=off  T_priority=None  T=0 K  T_nominal_specify=off  T_nominal_value=1  T_nominal_unit=K  Q_specify=off  Q_priority=None  Q=0 W  Q_nominal_specify=off  Q_nominal_value=1  Q_nominal_unit=W
  ar8 : fl_lib/Thermal/Thermal Elements/Convective Heat Transfer  thermal_type=foundation.enum.constant_variable.constant  area=pipeLenUFP*pipeHydrDiaUFP/2 m^2  heat_tr_coeff=htc W/(K*m^2)  min_heat_tr_coeff=1e-3 W/(K*m^2)  T_specify=off  T_priority=None  T=0 K  T_nominal_specify=off  T_nominal_value=1  T_nominal_unit=K  Q_specify=off  Q_priority=None  Q=0 W  Q_nominal_specify=off  Q_nominal_value=1  Q_nominal_unit=W
  V : PMIOPort  Side=Left
  S : PMIOPort  Port=2  Side=Left
  W4 : PMIOPort  Port=3  Side=Left
  TL_A : PMIOPort  Port=4  Side=Left
  W3 : PMIOPort  Port=5  Side=Left
  TL_B : PMIOPort  Port=6  Side=Right
  W2 : PMIOPort  Port=7  Side=Right
  T : PMIOPort  Port=8  Side=Right
  W1 : PMIOPort  Port=9  Side=Right
  Bottom : PMIOPort  Port=10  Side=Right
  Top : PMIOPort  Port=11  Side=Left
  connections:
  TL_B/RConn1 -- Room Underfloor Piping/RConn2 -- Room Wall Radiator/RConn2
  Room Volume1/RConn1 -- T/RConn1
  TL_A/RConn1 -- Room Underfloor Piping/LConn2 -- Room Wall Radiator/LConn2
  ar6/RConn1 -- W1/RConn1
  ar5/RConn1 -- W2/RConn1
  ar4/RConn1 -- W3/RConn1
  ar3/RConn1 -- W4/RConn1
  Thermal Resistance/LConn1 -- Room Underfloor Piping/RConn1 -- ar8/LConn1
  ar7/RConn1 -- Array Connection3/LConn2
  Top/RConn1 -- ar1/RConn1
  Thermal Resistance/RConn1 -- Bottom/RConn1
  Array Connection3/LConn3 -- ar3/LConn1
  Array Connection3/LConn4 -- ar4/LConn1
  Array Connection3/LConn5 -- ar5/LConn1
  Array Connection3/LConn6 -- ar6/LConn1
  Room Wall Radiator/RConn1 -- ar7/LConn1
  ar8/RConn1 -- Array Connection3/LConn1
  V/RConn1 -- PS Selector1/LConn1
  PS Selector1/RConn1 -- Room Underfloor Piping/LConn1 -- Room Wall Radiator/LConn1
  Room Volume1/LConn1 -- PS Selector/RConn1
  PS Selector/LConn1 -- S/RConn1
  Room Volume1/LConn3 -- Array Connection3/RConn1
  ar1/LConn1 -- Room Volume1/LConn2
